simulink model "Coupled_drives"  (R2019a)
settings: Solver=VariableStepAuto  StartTime=0.0  StopTime=200  RelTol=1e-3
settings Model: Creator=nbl  LastModifiedBy=alibei
settings DataIOCC: ReturnWorkspaceOutputs=off
settings DebuggingCC: PregeneratedLibrarySubsystemCodeDiagnostic=none  ArithmeticOperatorsInVariantConditions=warning
settings SFSimCC: SimUseLocalCustomCode=off
settings RTWCC: RTWUseLocalCustomCode=off

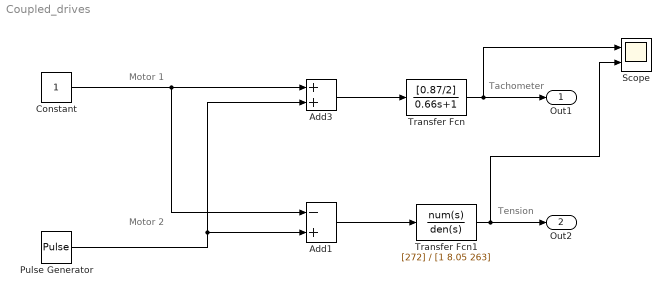
== system Coupled_drives ==
  note: Tension
  note: Tachometer
  note: Motor 1
  note: Motor 2
  Add1 : Sum  Inputs=-+
  Add3 : Sum  Inputs=2
  Constant : Constant
  Pulse Generator : DiscretePulseGenerator  PulseType=Time based  Period=50  PulseWidth=50
  Scope : Scope  NumInputPorts=2
  Transfer Fcn : TransferFcn  Numerator=[0.87/2]  Denominator=[0.66 1]
  Transfer Fcn1 : TransferFcn  Numerator=[272]  Denominator=[1 8.05 263]
  Out1 : Outport
  Out2 : Outport  Port=2
  wires:
  Add3/1 -> Transfer Fcn/1
  Add1/1 -> Transfer Fcn1/1
  Constant/1 -> Add1/1, Add3/1
  Pulse Generator/1 -> Add3/2, Add1/2
  Transfer Fcn/1 -> Scope/1, Out1/1
  Transfer Fcn1/1 -> Scope/2, Out2/1
